simulink model "Part_e"  (R2016a)
settings: Solver=VariableStepAuto  StartTime=0.0  StopTime=10.0  RelTol=1e-3
values from neighbouring files (symbols this model uses):
  A = [0 1 0 0 ... (first row only)    [Part_B.m]    (also in Part_C_D_E.m)
  Ao = A-L*C    [Part_C_D_E.m]
  B = [0;2*Calf/M;0;(2*Lf*Calf)/Iz]    [Part_B.m]    (also in Part_C_D_E.m)
  C = [0 0 1 0]    [Part_B.m]    (also in Part_C_D_E.m = [1 0 0 0])
  K = place(A,B,P)    [Part_C_D_E.m]
  L = place(A',C',P)'    [Part_C_D_E.m]
libraries: simulink x2
settings Model: Creator=ACER  LastModifiedBy=ACER

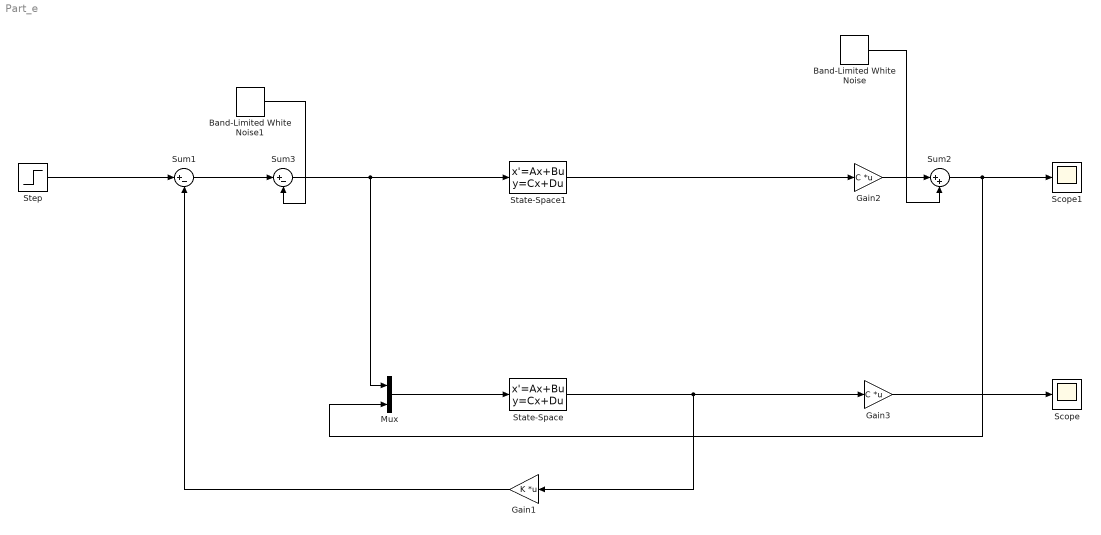
== system Part_e ==
  Band-Limited White Noise : simulink/Sources/Band-Limited White Noise  Cov=[0.1]  Ts=0.1  seed=[23341]
  Band-Limited White Noise1 : simulink/Sources/Band-Limited White Noise  Cov=[0.1]  Ts=0.1  seed=[23341]
  Gain1 : Gain  Gain=K  Multiplication=Matrix(K*u)
  Gain2 : Gain  Gain=C  Multiplication=Matrix(K*u)
  Gain3 : Gain  Gain=C  Multiplication=Matrix(K*u)
  Mux : Mux  Inputs=2
  Scope : Scope
  Scope1 : Scope
  State-Space : StateSpace  A=Ao  B=[B L]  C=eye(4)  D=[0 0;0 0;0 0;0 0]  X0=0
  State-Space1 : StateSpace  A=A  B=B  C=eye(4)  D=[0;0;0;0]  X0=0
  Step : Step  SampleTime=0
  Sum1 : Sum  Inputs=|+-
  Sum2 : Sum  Inputs=|++
  Sum3 : Sum  Inputs=|+-
  wires:
  Gain1/1 -> Sum1/2
  Step/1 -> Sum1/1
  Mux/1 -> State-Space/1
  State-Space1/1 -> Gain2/1
  State-Space/1 -> Gain3/1, Gain1/1
  Gain3/1 -> Scope/1
  Gain2/1 -> Sum2/1
  Sum2/1 -> Mux/2, Scope1/1
  Band-Limited White Noise/1 -> Sum2/2
  Sum3/1 -> Mux/1, State-Space1/1
  Band-Limited White Noise1/1 -> Sum3/2
  Sum1/1 -> Sum3/1
